simulink model "sim1_nonmininum_geso"  (R2018a)
settings: Solver=VariableStepAuto  StartTime=0.0  StopTime=60  RelTol=1e-3
values from neighbouring files (symbols this model uses):
  Ae = [Am,[0;1];[0 0 1]]    [ex1_liu_geso.m]
  Be = [Bm;0]    [ex1_liu_geso.m]
  Ce = [Cm,0]    [ex1_liu_geso.m]
  K0 = [K0b,1/nG(end)]    [ex1_liu_geso.m]
  L0 = fia*inv([Ce;Ce*Ae;Ce*Ae^2])*[0;0;1]    [ex1_liu_geso.m]
  Ts = 0.1    [ex1_liu.m]
libraries: cstblocks x5, simulink x1
settings Model: Creator=Bismark  LastModifiedBy=Bismark

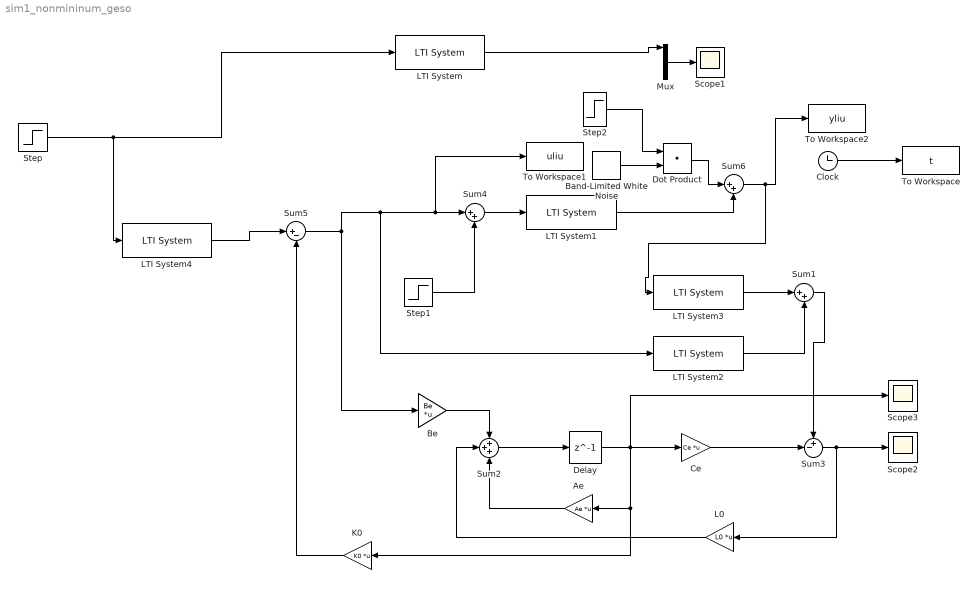
== system sim1_nonmininum_geso ==
  Ae : Gain  Gain=Ae  Multiplication=Matrix(K*u) (u vector)
  Band-Limited White Noise : simulink/Sources/Band-Limited White Noise  Cov=[0.00001]  Ts=Ts  seed=[23341]
  Be : Gain  Gain=Be  Multiplication=Matrix(K*u) (u vector)
  Ce : Gain  Gain=Ce  Multiplication=Matrix(K*u) (u vector)
  Clock : Clock
  Delay : Delay  DelayLength=1  SampleTime=Ts
  Dot Product : DotProduct  InputSameDT=on  OutDataTypeStr=Inherit: Inherit via internal rule
  K0 : Gain  Gain=K0  Multiplication=Matrix(K*u) (u vector)
  L0 : Gain  Gain=L0  Multiplication=Matrix(K*u) (u vector)
  LTI System : cstblocks/LTI System  sys=G  IC=[]
  LTI System1 : cstblocks/LTI System  sys=Pr  IC=[]
  LTI System2 : cstblocks/LTI System  sys=F1  IC=[]
  LTI System3 : cstblocks/LTI System  sys=F2  IC=[]
  LTI System4 : cstblocks/LTI System  sys=Kf  IC=[]
  Mux : Mux
  Scope1 : Scope
  Scope2 : Scope
  Scope3 : Scope
  Step : Step  Time=0  SampleTime=0
  Step1 : Step  Time=30  After=-1  SampleTime=Ts
  Step2 : Step  Time=55  SampleTime=0
  Sum1 : Sum  Inputs=|++
  Sum2 : Sum  Inputs=+++
  Sum3 : Sum  Inputs=+-|
  Sum4 : Sum  Inputs=|++
  Sum5 : Sum  Inputs=|+-
  Sum6 : Sum  Inputs=|++
  To Workspace : ToWorkspace  VariableName=t  SampleTime=Ts
  To Workspace1 : ToWorkspace  VariableName=uliu  SampleTime=Ts
  To Workspace2 : ToWorkspace  VariableName=yliu  SampleTime=Ts
  wires:
  Sum5/1 -> LTI System2/1, To Workspace1/1, Sum4/1, Be/1
  LTI System/1 -> Mux/1
  Mux/1 -> Scope1/1
  Clock/1 -> To Workspace/1
  Sum4/1 -> LTI System1/1
  Step1/1 -> Sum4/2
  LTI System3/1 -> Sum1/1
  LTI System2/1 -> Sum1/2
  Sum1/1 -> Sum3/1
  Be/1 -> Sum2/1
  Sum2/1 -> Delay/1
  Delay/1 -> Scope3/1, K0/1, Ae/1, Ce/1
  Ce/1 -> Sum3/2
  Ae/1 -> Sum2/3
  Sum3/1 -> Scope2/1, L0/1
  L0/1 -> Sum2/2
  LTI System4/1 -> Sum5/1
  Step/1 -> LTI System4/1, LTI System/1
  K0/1 -> Sum5/2
  Step2/1 -> Dot Product/1
  Band-Limited White Noise/1 -> Dot Product/2
  LTI System1/1 -> Sum6/2
  Sum6/1 -> LTI System3/1, To Workspace2/1
  Dot Product/1 -> Sum6/1
